simulink model "BVH2_App_Layer"  (Simulink 5.1)
settings: Solver=ode45  StartTime=0.0  StopTime=10.0  RelTol=1e-3
PreLoadFcn:
  | if exist('tl_preloadfcn','file'), tl_preloadfcn(gcs,95); end
PostLoadFcn:
  | if exist('tl_postloadfcn','file'), tl_postloadfcn(gcs,95); end
InitFcn:
  | if exist('tlds_start','file'), tlds_start(gcs); end
undefined symbols (not defined in the file): built, constant, Constant, DiscreteIntegrator, Gain, in, Logic, Product, Saturate, Sum, Switch
libraries: tllib x71, simulink x1
(part 2 of 4)

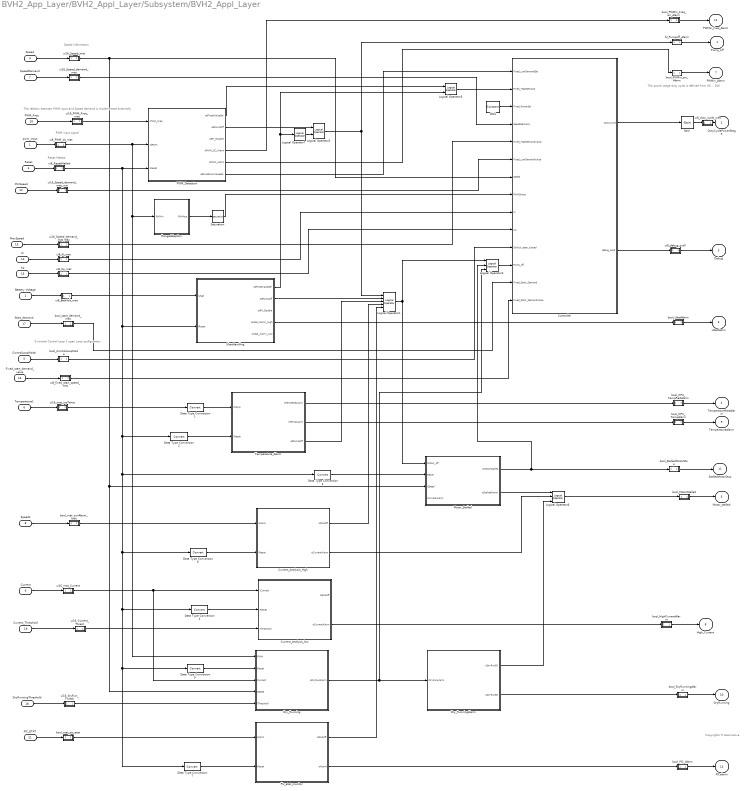
== system BVH2_App_Layer/BVH2_Appl_Layer/Subsystem/BVH2_Appl_Layer ==
  note: Copyrights
      | TI Automotive
  note: The power stage duty cycle
      | is defined from 00 .. 200
  note: 0   normal Control Loop
      | 1 open Loop configuration
  note: The relation between PWM input
      | and Speed demand is implemented externally
  note: Speed information
  note: PWM input signal
  note: Reset Matlab
  pwm_input : Inport  PortDimensions=1  SampleTime=0.01
      settings: CopyFcn=if exist('tl_check_ports','file'), tl_check_ports(gcbh); end  NameChangeFcn=if exist('tl_check_ports','file'), tl_check_ports(gcbh); end
  Battery Voltage : Inport  Port=2  PortDimensions=1  SampleTime=0.01
      settings: CopyFcn=if exist('tl_check_ports','file'), tl_check_ports(gcbh); end  NameChangeFcn=if exist('tl_check_ports','file'), tl_check_ports(gcbh); end
  Reset : Inport  Port=3  SampleTime=0.01
      settings: CopyFcn=if exist('tl_check_ports','file'), tl_check_ports(gcbh); end  NameChangeFcn=if exist('tl_check_ports','file'), tl_check_ports(gcbh); end
  Speed : Inport  Port=4  PortDimensions=1  SampleTime=0.01
      settings: CopyFcn=if exist('tl_check_ports','file'), tl_check_ports(gcbh); end  NameChangeFcn=if exist('tl_check_ports','file'), tl_check_ports(gcbh); end
  ControlLoopMode : Inport  Port=5  PortDimensions=1  SampleTime=0.01
      settings: CopyFcn=if exist('tl_check_ports','file'), tl_check_ports(gcbh); end  NameChangeFcn=if exist('tl_check_ports','file'), tl_check_ports(gcbh); end
  Temperature1 : Inport  Port=6  PortDimensions=1  SampleTime=0.01
      settings: CopyFcn=if exist('tl_check_ports','file'), tl_check_ports(gcbh); end  NameChangeFcn=if exist('tl_check_ports','file'), tl_check_ports(gcbh); end
  SpeedDemand : Inport  Port=7  PortDimensions=1  SampleTime=0.01
      settings: CopyFcn=if exist('tl_check_ports','file'), tl_check_ports(gcbh); end  NameChangeFcn=if exist('tl_check_ports','file'), tl_check_ports(gcbh); end
  Speed1 : Inport  Port=8  PortDimensions=1  SampleTime=0.01
      settings: CopyFcn=if exist('tl_check_ports','file'), tl_check_ports(gcbh); end  NameChangeFcn=if exist('tl_check_ports','file'), tl_check_ports(gcbh); end
  Current : Inport  Port=9  PortDimensions=1  SampleTime=0.01
      settings: CopyFcn=if exist('tl_check_ports','file'), tl_check_ports(gcbh); end  NameChangeFcn=if exist('tl_check_ports','file'), tl_check_ports(gcbh); end
  PWM_Freq : Inport  Port=10  PortDimensions=1  SampleTime=0.01
      settings: CopyFcn=if exist('tl_check_ports','file'), tl_check_ports(gcbh); end  NameChangeFcn=if exist('tl_check_ports','file'), tl_check_ports(gcbh); end
  PIC_ETAT : Inport  Port=11  PortDimensions=1  SampleTime=0.01
      settings: CopyFcn=if exist('tl_check_ports','file'), tl_check_ports(gcbh); end  NameChangeFcn=if exist('tl_check_ports','file'), tl_check_ports(gcbh); end
  MinSpeed : Inport  Port=12  SampleTime=0.01
      settings: CopyFcn=if exist('tl_check_ports','file'), tl_check_ports(gcbh); end  NameChangeFcn=if exist('tl_check_ports','file'), tl_check_ports(gcbh); end
  MaxSpeed : Inport  Port=13  SampleTime=0.01
      settings: CopyFcn=if exist('tl_check_ports','file'), tl_check_ports(gcbh); end  NameChangeFcn=if exist('tl_check_ports','file'), tl_check_ports(gcbh); end
  Ki : Inport  Port=14  SampleTime=0.01
      settings: CopyFcn=if exist('tl_check_ports','file'), tl_check_ports(gcbh); end  NameChangeFcn=if exist('tl_check_ports','file'), tl_check_ports(gcbh); end
  Kp : Inport  Port=15  SampleTime=0.01
      settings: CopyFcn=if exist('tl_check_ports','file'), tl_check_ports(gcbh); end  NameChangeFcn=if exist('tl_check_ports','file'), tl_check_ports(gcbh); end
  Fixed_start_demand_value : Inport  Port=16  PortDimensions=1  SampleTime=0.01
      settings: CopyFcn=if exist('tl_check_ports','file'), tl_check_ports(gcbh); end  NameChangeFcn=if exist('tl_check_ports','file'), tl_check_ports(gcbh); end
  Start_demand : Inport  Port=17  PortDimensions=1  SampleTime=0.01
      settings: CopyFcn=if exist('tl_check_ports','file'), tl_check_ports(gcbh); end  NameChangeFcn=if exist('tl_check_ports','file'), tl_check_ports(gcbh); end
  DryRunningThreshold : Inport  Port=18  PortDimensions=1  SampleTime=0.01
      settings: CopyFcn=if exist('tl_check_ports','file'), tl_check_ports(gcbh); end  NameChangeFcn=if exist('tl_check_ports','file'), tl_check_ports(gcbh); end
  Current_Threshold : Inport  Port=19  PortDimensions=1  SampleTime=0.01
      settings: CopyFcn=if exist('tl_check_ports','file'), tl_check_ports(gcbh); end  NameChangeFcn=if exist('tl_check_ports','file'), tl_check_ports(gcbh); end
  Controller : Subsystem
  Current_Analysis_High : Stateflow chart
  Current_Analysis_low : Stateflow chart
  Data Type Conversion{1..7} (7 alike) : DataTypeConversion  SaturateOnIntegerOverflow=on
  Dry_Running : Stateflow chart
  Dry_RunningAlarm : Stateflow chart
  Gain : tllib/Gain  data=struct('comment',struct('text','','placement',1),'logdata',struct('maxnumvals',inf,'plotchannels',[],'loggingmode',3,'channels',1),'output',struct('variable','','description','','name','$S_$B','width',1,'address','','max',NaN,'min',NaN,'class','default','type','Int16','scaling','','lsb',1,'offset',0,'arb',0,'freeze',1,'unit','','autoscalingmode',1,'lowerheadroom',1,'upperheadroom',1,'headroomunit','bit','keepdatatype',1,'checkmin',0,'checkmax',0,'castoutput',0,'show',0),'gain',struct('variable','','description','','name','$S_$B_gain','width',1,'address','','max',NaN,'min',NaN,'class','default','type','Int16','scaling','','lsb',1,'offset',0,'arb',0,'freeze',1,'unit','','keepdatatype',1,'value','0.5','scalar',0,'tolerance',1),'scalingvalid',0,'date',734649.702698634)  gain=0.5  flp_block=built-in/Gain
  Logical Operator1 : tllib/Logical Operator  data=struct('inputs','5','comment',struct('text','','placement',1),'logdata',struct('maxnumvals',inf,'plotchannels',[],'loggingmode',3,'channels',1),'operator','OR','output',struct('variable','','description','','name','$S_$B','address','','class','default','type','Bool','unit',''),'scalingvalid',0,'date',736089.717150243)  flp_block=built-in/Logic
  Logical Operator2 : tllib/Logical Operator  data=struct('inputs','2','comment',struct('text','','placement',1),'logdata',struct('maxnumvals',inf,'plotchannels',[],'loggingmode',3,'channels',1),'operator','AND','output',struct('variable','','description','','name','$S_$B','address','','class','default','type','Bool','unit',''),'scalingvalid',0,'date',735166.438757674)  flp_block=built-in/Logic
  Logical Operator3 : tllib/Logical Operator  data=struct('inputs','3','comment',struct('text','','placement',1),'logdata',struct('maxnumvals',inf,'plotchannels',[],'loggingmode',3,'channels',1),'operator','OR','output',struct('variable','','description','','name','$S_$B','address','','class','default','type','Bool','unit',''),'scalingvalid',0,'date',736089.716464456)  flp_block=built-in/Logic
  Logical Operator5 : tllib/Logical Operator  data=struct('inputs','2','comment',struct('text','','placement',1),'logdata',struct('maxnumvals',inf,'plotchannels',[],'loggingmode',3,'channels',1),'operator','OR','output',struct('variable','','description','','name','$S_$B','address','','class','default','type','Bool','unit',''),'scalingvalid',0,'date',735166.427160579)  flp_block=built-in/Logic
  Logical Operator6 : tllib/Logical Operator  data=struct('inputs','3','comment',struct('text','','placement',1),'logdata',struct('maxnumvals',inf,'plotchannels',[],'loggingmode',3,'channels',1),'operator','OR','output',struct('variable','','description','','name','$S_$B','address','','class','default','type','Bool','unit',''),'scalingvalid',0,'date',736074.585590822)  flp_block=built-in/Logic
  Logical Operator7 : tllib/Logical Operator  data=struct('inputs','1','comment',struct('text','','placement',1),'logdata',struct('maxnumvals',inf,'plotchannels',[],'loggingmode',3,'channels',1),'operator','NOT','output',struct('variable','','description','','name','$S_$B','address','','class','default','type','Bool','unit',''),'scalingvalid',0,'date',735166.438991285)  flp_block=built-in/Logic
  Motor_Stalled : Stateflow chart
  ON4 : tllib/Constant  Value=constant  ShowAdditionalParam=off  OutDataType=sfix(16)  ConRadixGroup=Use specified scaling  OutScaling=2^0  data=struct('comment',struct('text','','placement',1),'output',struct('width',1,'name','$S_$B','unit','','type','Int16','offset',0,'max',NaN,'min',NaN,'freeze',1,'lsb',1,'arb',0,'class','default','address','','description','','value','0','tolerance',1,'show',0,'variable','','scaling','','keepdatatype',1),'date',734769.5812564,'scalingvalid',0)  constant=0  flp_block=built-in/Constant  help=|
      | Constant block of dSPACE TargetLink.
      | 
      | Output signal keeps the given constant value.
  PWM_Detection : Stateflow chart
  Pic_etat_monitor : Stateflow chart
  RangeAdaption : Subsystem
  Saturation : tllib/Saturation  data=struct('comment',struct('text','','placement',1),'logdata',struct('maxnumvals',inf,'plotchannels',[],'loggingmode',3,'channels',1),'output',struct('variable','','description','','name','$S_$B','width',1,'address','','max',NaN,'min',NaN,'class','default','type','UInt8','scaling','','lsb',1,'offset',0,'arb',0,'freeze',1,'unit','','autoscalingmode',1,'lowerheadroom',0,'upperheadroom',1,'headroomunit','bit','keepdatatype',1,'castoutput',0,'show',0),'lowerlimit',struct('variable','','description','','name','$S_$B_lower','width',1,'address','','max',NaN,'min',NaN,'class','default','type','Int16','scaling','','lsb',1,'offset',0,'arb',0,'freeze',1,'unit','','keepdatatype',1,'value','60','scalar',0),'upperlimit',struct('variable','','description','','name','$S_$B_upper','width',1,'address','','max',NaN,'min',NaN,'class','default','type','Int16','scaling','','lsb',1,'offset',0,'arb',0,'freeze',1,'unit','','keepdatatype',1,'value','200','scalar',0),'scalingvalid',0,'date',734975.431625949)  lower_limit=60  upper_limit=200  flp_block=built-in/Saturate
  Temperature_Alarm : Stateflow chart
  UbatHandling : Stateflow chart
  bl_Pumpoff_Alarm : Subsystem  BlockChoice=Virtual  mask(TL_Outport){data=struct('comment',struct('text','','placement',1),'logdata',struct('maxnumvals',inf,'plotchannels',[],'loggingmode',3,'channels',1),'output',struct('width',1,'name','$B','unit','','type','Bool','offset',0,'max',NaN,'min',NaN,'freeze',1,'lsb',1,'arb',0,'class','GLOBAL','address','','description','','autoscalingmode',1,'lowerheadroom',0,'upperheadroom',1,'headroomunit','bit','checkmin',0,'checkmax',0,'show',0,'variable','','scaling','','keepdatatype',1,'castoutput',0),'date',734767.568817153,'message',struct('name','','component',''),'virtual',1,'scalingvalid',0), flp_block=none, slscaleparams=, help=|}
      mask help=|
      | OutPort block of dSPACE TargetLink.
      |
      | Input signal is scaled:
      |
      |         y = lsb * u + offset
      mask help:
      | TargetLink Outport block:
      | Defines the output interface of a TargetLink subsystem.
      mask init:
      | tlData = eval(data);
      | w = tlData.output.width;
      | if ~isempty(tlData.output.variable)
      |    [bExist,hVar] = dsdd('Exist',['/Pool/Variables/' tlData.output.variable],'ObjectKind','Variable');
      |    if bExist,
      |       w = dsdd('GetWidth',hVar);
      |       if isempty(w)
      |          w = 1;
      |       end
      |    end
      | end
      | if ~strcmp(get_param(gcbh,'TemplateBlock'),'')
      |    if tlData.virtual,
      |       if tlData.logdata.loggingmode == 3
      |          set_param(gcbh,'BlockChoice','Virtual');
      |       else
      |          set_param(gcbh,'BlockChoice','Mixed');
      |       end
      |    else
      |       set_param(gcbh,'BlockChoice','NonVirtual');
      |    end
      | end
      | clear tlData
      settings: DeleteFcn=delete_tlblock(gcbh);  NameChangeFcn=rename_tlblock(gcbh);  OpenFcn=dstabdlg('create','tl_port_dlg',gcbh);  TemplateBlock=tllib/OutPort  MemberBlocks=Mixed,NonVirtual,Virtual
      mask Help: eval(['tl_online_help(''Topic'',''',get_param(gcbh,'MaskType'),''')'])
      mask Display: plot([0 .2 .2 .8 .8; 1 .8 .8 .8 .8],[.5 .6 .4 .6 .4;.5 .6 .4 .8 .2]);
  bool_CPU_TempAlarm : Subsystem  BlockChoice=Virtual  mask(TL_Outport){data=struct('comment',struct('text','','placement',1),'logdata',struct('maxnumvals',inf,'plotchannels',[],'loggingmode',3,'channels',1),'output',struct('width',1,'name','$B','unit','','type','Bool','offset',0,'max',NaN,'min',NaN,'freeze',1,'lsb',1,'arb',0,'class','GLOBAL','address','','description','','autoscalingmode',1,'lowerheadroom',0,'upperheadroom',1,'headroomunit','bit','checkmin',0,'checkmax',0,'show',0,'variable','','scaling','','keepdatatype',1,'castoutput',0),'date',734773.577754271,'message',struct('name','','component',''),'virtual',1,'scalingvalid',0), flp_block=none, slscaleparams=, help=|}
      mask help=|
      | OutPort block of dSPACE TargetLink.
      |
      | Input signal is scaled:
      |
      |         y = lsb * u + offset
      mask help:
      | TargetLink Outport block:
      | Defines the output interface of a TargetLink subsystem.
      mask init: same as BVH2_App_Layer/BVH2_Appl_Layer/Subsystem/BVH2_Appl_Layer/bl_Pumpoff_Alarm
      settings: DeleteFcn=delete_tlblock(gcbh);  NameChangeFcn=rename_tlblock(gcbh);  OpenFcn=dstabdlg('create','tl_port_dlg',gcbh);  TemplateBlock=tllib/OutPort  MemberBlocks=Mixed,NonVirtual,Virtual
      mask Help: eval(['tl_online_help(''Topic'',''',get_param(gcbh,'MaskType'),''')'])
      mask Display: plot([0 .2 .2 .8 .8; 1 .8 .8 .8 .8],[.5 .6 .4 .6 .4;.5 .6 .4 .8 .2]);
  bool_CPU_TempRedAlarm : Subsystem  BlockChoice=Virtual  mask(TL_Outport){data=struct('comment',struct('text','','placement',1),'logdata',struct('maxnumvals',inf,'plotchannels',[],'loggingmode',3,'channels',1),'output',struct('width',1,'name','$B','unit','','type','Bool','offset',0,'max',NaN,'min',NaN,'freeze',1,'lsb',1,'arb',0,'class','GLOBAL','address','','description','','autoscalingmode',1,'lowerheadroom',0,'upperheadroom',1,'headroomunit','bit','checkmin',0,'checkmax',0,'show',0,'variable','','scaling','','keepdatatype',1,'castoutput',0),'date',734773.577754271,'message',struct('name','','component',''),'virtual',1,'scalingvalid',0), flp_block=none, slscaleparams=, help=|}
      mask help=|
      | OutPort block of dSPACE TargetLink.
      |
      | Input signal is scaled:
      |
      |         y = lsb * u + offset
      mask help:
      | TargetLink Outport block:
      | Defines the output interface of a TargetLink subsystem.
      mask init: same as BVH2_App_Layer/BVH2_Appl_Layer/Subsystem/BVH2_Appl_Layer/bl_Pumpoff_Alarm
      settings: DeleteFcn=delete_tlblock(gcbh);  NameChangeFcn=rename_tlblock(gcbh);  OpenFcn=dstabdlg('create','tl_port_dlg',gcbh);  TemplateBlock=tllib/OutPort  MemberBlocks=Mixed,NonVirtual,Virtual
      mask Help: eval(['tl_online_help(''Topic'',''',get_param(gcbh,'MaskType'),''')'])
      mask Display: plot([0 .2 .2 .8 .8; 1 .8 .8 .8 .8],[.5 .6 .4 .6 .4;.5 .6 .4 .8 .2]);
  bool_ControlLoopMode : Subsystem  BlockChoice=Mixed  mask(TL_Inport){data=struct('logdata',struct('maxnumvals',inf,'plotchannels',1,'loggingmode',1,'channels',1),'output',struct('width',1,'name','$B','unit','','type','Bool','offset',0,'max',NaN,'min',NaN,'freeze',1,'lsb',1,'arb',0,'class','GLOBAL','address','','description','','autoscalingmode',1,'lowerheadroom',0,'upperheadroom',1,'headroomunit','bit','show',0,'variable','','scaling','','keepdatatype',1,'castoutput',0),'date',734773.443896898,'message',struct('name','','component','','accessor',''),'virtual',1,'scalingvalid',0), flp_block=none, slscaleparams=, help=|}
      mask help=|
      | InPort block of dSPACE TargetLink.
      |
      | Input signal is read from an external variable and scaled:
      |
      |         y = lsb * u + offset
      mask help:
      | TargetLink Inport block:
      | Defines the input interface of a TargetLink subsystem.
      mask init: same as BVH2_App_Layer/BVH2_Appl_Layer/Subsystem/BVH2_Appl_Layer/bl_Pumpoff_Alarm
      settings: DeleteFcn=delete_tlblock(gcbh);  NameChangeFcn=rename_tlblock(gcbh);  OpenFcn=dstabdlg('create','tl_port_dlg',gcbh);  TemplateBlock=tllib/InPort  MemberBlocks=Mixed,NonVirtual,Virtual
      mask Help: eval(['tl_online_help(''Topic'',''',get_param(gcbh,'MaskType'),''')'])
      mask Display: plot([.2 0 .2 .2 .2;.2 1 .8 .8 .2],[.8 .5 .6 .4 .2;.6 .5 .6 .4 .4]);
  bool_DryRunningAlarm : Subsystem  BlockChoice=Virtual  mask(TL_Outport){data=struct('comment',struct('text','','placement',1),'logdata',struct('maxnumvals',inf,'plotchannels',[],'loggingmode',3,'channels',1),'output',struct('width',1,'name','$B','unit','','type','Bool','offset',0,'max',NaN,'min',NaN,'freeze',1,'lsb',1,'arb',0,'class','GLOBAL','address','','description','','autoscalingmode',1,'lowerheadroom',0,'upperheadroom',1,'headroomunit','bit','checkmin',0,'checkmax',0,'show',0,'variable','','scaling','','keepdatatype',1,'castoutput',0),'date',734773.60810485,'message',struct('name','','component',''),'virtual',1,'scalingvalid',0), flp_block=none, slscaleparams=, help=|}
      mask help=|
      | OutPort block of dSPACE TargetLink.
      |
      | Input signal is scaled:
      |
      |         y = lsb * u + offset
      mask help:
      | TargetLink Outport block:
      | Defines the output interface of a TargetLink subsystem.
      mask init: same as BVH2_App_Layer/BVH2_Appl_Layer/Subsystem/BVH2_Appl_Layer/bl_Pumpoff_Alarm
      settings: DeleteFcn=delete_tlblock(gcbh);  NameChangeFcn=rename_tlblock(gcbh);  OpenFcn=dstabdlg('create','tl_port_dlg',gcbh);  TemplateBlock=tllib/OutPort  MemberBlocks=Mixed,NonVirtual,Virtual
      mask Help: eval(['tl_online_help(''Topic'',''',get_param(gcbh,'MaskType'),''')'])
      mask Display: plot([0 .2 .2 .8 .8; 1 .8 .8 .8 .8],[.5 .6 .4 .6 .4;.5 .6 .4 .8 .2]);
  bool_HighCurrentAlarm : Subsystem  BlockChoice=Virtual  mask(TL_Outport){data=struct('comment',struct('text','','placement',1),'logdata',struct('maxnumvals',inf,'plotchannels',[],'loggingmode',3,'channels',1),'output',struct('width',1,'name','$B','unit','','type','Bool','offset',0,'max',NaN,'min',NaN,'freeze',1,'lsb',1,'arb',0,'class','GLOBAL','address','','description','','autoscalingmode',1,'lowerheadroom',0,'upperheadroom',1,'headroomunit','bit','checkmin',0,'checkmax',0,'show',0,'variable','','scaling','','keepdatatype',1,'castoutput',0),'date',734773.60810485,'message',struct('name','','component',''),'virtual',1,'scalingvalid',0), flp_block=none, slscaleparams=, help=|}
      mask help=|
      | OutPort block of dSPACE TargetLink.
      |
      | Input signal is scaled:
      |
      |         y = lsb * u + offset
      mask help:
      | TargetLink Outport block:
      | Defines the output interface of a TargetLink subsystem.
      mask init: same as BVH2_App_Layer/BVH2_Appl_Layer/Subsystem/BVH2_Appl_Layer/bl_Pumpoff_Alarm
      settings: DeleteFcn=delete_tlblock(gcbh);  NameChangeFcn=rename_tlblock(gcbh);  OpenFcn=dstabdlg('create','tl_port_dlg',gcbh);  TemplateBlock=tllib/OutPort  MemberBlocks=Mixed,NonVirtual,Virtual
      mask Help: eval(['tl_online_help(''Topic'',''',get_param(gcbh,'MaskType'),''')'])
      mask Display: plot([0 .2 .2 .8 .8; 1 .8 .8 .8 .8],[.5 .6 .4 .6 .4;.5 .6 .4 .8 .2]);
  bool_MotorStalled : Subsystem  BlockChoice=Virtual  mask(TL_Outport){data=struct('comment',struct('text','','placement',1),'logdata',struct('maxnumvals',inf,'plotchannels',[],'loggingmode',3,'channels',1),'output',struct('width',1,'name','$B','unit','','type','Bool','offset',0,'max',NaN,'min',NaN,'freeze',1,'lsb',1,'arb',0,'class','GLOBAL','address','','description','','autoscalingmode',1,'lowerheadroom',0,'upperheadroom',1,'headroomunit','bit','checkmin',0,'checkmax',0,'show',0,'variable','','scaling','','keepdatatype',1,'castoutput',0),'date',734773.60810485,'message',struct('name','','component',''),'virtual',1,'scalingvalid',0), flp_block=none, slscaleparams=, help=|}
      mask help=|
      | OutPort block of dSPACE TargetLink.
      |
      | Input signal is scaled:
      |
      |         y = lsb * u + offset
      mask help:
      | TargetLink Outport block:
      | Defines the output interface of a TargetLink subsystem.
      mask init: same as BVH2_App_Layer/BVH2_Appl_Layer/Subsystem/BVH2_Appl_Layer/bl_Pumpoff_Alarm
      settings: DeleteFcn=delete_tlblock(gcbh);  NameChangeFcn=rename_tlblock(gcbh);  OpenFcn=dstabdlg('create','tl_port_dlg',gcbh);  TemplateBlock=tllib/OutPort  MemberBlocks=Mixed,NonVirtual,Virtual
      mask Help: eval(['tl_online_help(''Topic'',''',get_param(gcbh,'MaskType'),''')'])
      mask Display: plot([0 .2 .2 .8 .8; 1 .8 .8 .8 .8],[.5 .6 .4 .6 .4;.5 .6 .4 .8 .2]);
  bool_PIC_Alarm : Subsystem  BlockChoice=Virtual  mask(TL_Outport){data=struct('comment',struct('text','','placement',1),'logdata',struct('maxnumvals',inf,'plotchannels',[],'loggingmode',3,'channels',1),'output',struct('width',1,'name','$B','unit','','type','Bool','offset',0,'max',NaN,'min',NaN,'freeze',1,'lsb',1,'arb',0,'class','GLOBAL','address','','description','','autoscalingmode',1,'lowerheadroom',0,'upperheadroom',1,'headroomunit','bit','checkmin',0,'checkmax',0,'show',0,'variable','','scaling','','keepdatatype',1,'castoutput',0),'date',734773.60810485,'message',struct('name','','component',''),'virtual',1,'scalingvalid',0), flp_block=none, slscaleparams=, help=|}
      mask help=|
      | OutPort block of dSPACE TargetLink.
      |
      | Input signal is scaled:
      |
      |         y = lsb * u + offset
      mask help:
      | TargetLink Outport block:
      | Defines the output interface of a TargetLink subsystem.
      mask init: same as BVH2_App_Layer/BVH2_Appl_Layer/Subsystem/BVH2_Appl_Layer/bl_Pumpoff_Alarm
      settings: DeleteFcn=delete_tlblock(gcbh);  NameChangeFcn=rename_tlblock(gcbh);  OpenFcn=dstabdlg('create','tl_port_dlg',gcbh);  TemplateBlock=tllib/OutPort  MemberBlocks=Mixed,NonVirtual,Virtual
      mask Help: eval(['tl_online_help(''Topic'',''',get_param(gcbh,'MaskType'),''')'])
      mask Display: plot([0 .2 .2 .8 .8; 1 .8 .8 .8 .8],[.5 .6 .4 .6 .4;.5 .6 .4 .8 .2]);
  bool_PWMin_Freq_err_Alarm : Subsystem  BlockChoice=Virtual  mask(TL_Outport){data=struct('comment',struct('text','','placement',1),'logdata',struct('maxnumvals',inf,'plotchannels',[],'loggingmode',3,'channels',1),'output',struct('width',1,'name','$B','unit','','type','Bool','offset',0,'max',NaN,'min',NaN,'freeze',1,'lsb',1,'arb',0,'class','GLOBAL','address','','description','','autoscalingmode',1,'lowerheadroom',0,'upperheadroom',1,'headroomunit','bit','checkmin',0,'checkmax',0,'show',0,'variable','','scaling','','keepdatatype',1,'castoutput',0),'date',734767.568817153,'message',struct('name','','component',''),'virtual',1,'scalingvalid',0), flp_block=none, slscaleparams=, help=|}
      mask help=|
      | OutPort block of dSPACE TargetLink.
      |
      | Input signal is scaled:
      |
      |         y = lsb * u + offset
      mask help:
      | TargetLink Outport block:
      | Defines the output interface of a TargetLink subsystem.
      mask init: same as BVH2_App_Layer/BVH2_Appl_Layer/Subsystem/BVH2_Appl_Layer/bl_Pumpoff_Alarm
      settings: DeleteFcn=delete_tlblock(gcbh);  NameChangeFcn=rename_tlblock(gcbh);  OpenFcn=dstabdlg('create','tl_port_dlg',gcbh);  TemplateBlock=tllib/OutPort  MemberBlocks=Mixed,NonVirtual,Virtual
      mask Help: eval(['tl_online_help(''Topic'',''',get_param(gcbh,'MaskType'),''')'])
      mask Display: plot([0 .2 .2 .8 .8; 1 .8 .8 .8 .8],[.5 .6 .4 .6 .4;.5 .6 .4 .8 .2]);
  bool_PWMin_err_Alarm : Subsystem  BlockChoice=Virtual  mask(TL_Outport){data=struct('comment',struct('text','','placement',1),'logdata',struct('maxnumvals',inf,'plotchannels',[],'loggingmode',3,'channels',1),'output',struct('width',1,'name','$B','unit','','type','Bool','offset',0,'max',NaN,'min',NaN,'freeze',1,'lsb',1,'arb',0,'class','GLOBAL','address','','description','','autoscalingmode',1,'lowerheadroom',0,'upperheadroom',1,'headroomunit','bit','checkmin',0,'checkmax',0,'show',0,'variable','','scaling','','keepdatatype',1,'castoutput',0),'date',734767.568817153,'message',struct('name','','component',''),'virtual',1,'scalingvalid',0), flp_block=none, slscaleparams=, help=|}
      mask help=|
      | OutPort block of dSPACE TargetLink.
      |
      | Input signal is scaled:
      |
      |         y = lsb * u + offset
      mask help:
      | TargetLink Outport block:
      | Defines the output interface of a TargetLink subsystem.
      mask init: same as BVH2_App_Layer/BVH2_Appl_Layer/Subsystem/BVH2_Appl_Layer/bl_Pumpoff_Alarm
      settings: DeleteFcn=delete_tlblock(gcbh);  NameChangeFcn=rename_tlblock(gcbh);  OpenFcn=dstabdlg('create','tl_port_dlg',gcbh);  TemplateBlock=tllib/OutPort  MemberBlocks=Mixed,NonVirtual,Virtual
      mask Help: eval(['tl_online_help(''Topic'',''',get_param(gcbh,'MaskType'),''')'])
      mask Display: plot([0 .2 .2 .8 .8; 1 .8 .8 .8 .8],[.5 .6 .4 .6 .4;.5 .6 .4 .8 .2]);
  bool_StalledMotorStop : Subsystem  BlockChoice=Virtual  mask(TL_Outport){data=struct('comment',struct('text','','placement',1),'logdata',struct('maxnumvals',inf,'plotchannels',[],'loggingmode',3,'channels',1),'output',struct('width',1,'name','$B','unit','','type','Bool','offset',0,'max',NaN,'min',NaN,'freeze',1,'lsb',1,'arb',0,'class','GLOBAL','address','','description','','autoscalingmode',1,'lowerheadroom',0,'upperheadroom',1,'headroomunit','bit','checkmin',0,'checkmax',0,'show',0,'variable','','scaling','','keepdatatype',1,'castoutput',0),'date',734773.60810485,'message',struct('name','','component',''),'virtual',1,'scalingvalid',0), flp_block=none, slscaleparams=, help=|}
      mask help=|
      | OutPort block of dSPACE TargetLink.
      |
      | Input signal is scaled:
      |
      |         y = lsb * u + offset
      mask help:
      | TargetLink Outport block:
      | Defines the output interface of a TargetLink subsystem.
      mask init: same as BVH2_App_Layer/BVH2_Appl_Layer/Subsystem/BVH2_Appl_Layer/bl_Pumpoff_Alarm
      settings: DeleteFcn=delete_tlblock(gcbh);  NameChangeFcn=rename_tlblock(gcbh);  OpenFcn=dstabdlg('create','tl_port_dlg',gcbh);  TemplateBlock=tllib/OutPort  MemberBlocks=Mixed,NonVirtual,Virtual
      mask Help: eval(['tl_online_help(''Topic'',''',get_param(gcbh,'MaskType'),''')'])
      mask Display: plot([0 .2 .2 .8 .8; 1 .8 .8 .8 .8],[.5 .6 .4 .6 .4;.5 .6 .4 .8 .2]);
  bool_UbatAlarm : Subsystem  BlockChoice=Virtual  mask(TL_Outport){data=struct('comment',struct('text','','placement',1),'logdata',struct('maxnumvals',inf,'plotchannels',[],'loggingmode',3,'channels',1),'output',struct('width',1,'name','$B','unit','','type','Bool','offset',0,'max',NaN,'min',NaN,'freeze',1,'lsb',1,'arb',0,'class','GLOBAL','address','','description','','autoscalingmode',1,'lowerheadroom',0,'upperheadroom',1,'headroomunit','bit','checkmin',0,'checkmax',0,'show',0,'variable','','scaling','','keepdatatype',1,'castoutput',0),'date',734767.568817153,'message',struct('name','','component',''),'virtual',1,'scalingvalid',0), flp_block=none, slscaleparams=, help=|}
      mask help=|
      | OutPort block of dSPACE TargetLink.
      |
      | Input signal is scaled:
      |
      |         y = lsb * u + offset
      mask help:
      | TargetLink Outport block:
      | Defines the output interface of a TargetLink subsystem.
      mask init: same as BVH2_App_Layer/BVH2_Appl_Layer/Subsystem/BVH2_Appl_Layer/bl_Pumpoff_Alarm
      settings: DeleteFcn=delete_tlblock(gcbh);  NameChangeFcn=rename_tlblock(gcbh);  OpenFcn=dstabdlg('create','tl_port_dlg',gcbh);  TemplateBlock=tllib/OutPort  MemberBlocks=Mixed,NonVirtual,Virtual
      mask Help: eval(['tl_online_help(''Topic'',''',get_param(gcbh,'MaskType'),''')'])
      mask Display: plot([0 .2 .2 .8 .8; 1 .8 .8 .8 .8],[.5 .6 .4 .6 .4;.5 .6 .4 .8 .2]);
  bool_mat_currAlarm_bldc : Subsystem  BlockChoice=Mixed  mask(TL_Inport){data=struct('logdata',struct('maxnumvals',inf,'plotchannels',1,'loggingmode',1,'channels',1),'output',struct('width',1,'name','$B','unit','','type','Bool','offset',0,'max',NaN,'min',NaN,'freeze',1,'lsb',1,'arb',0,'class','GLOBAL','address','','description','','autoscalingmode',1,'lowerheadroom',0,'upperheadroom',1,'headroomunit','bit','show',0,'variable','','scaling','','keepdatatype',1,'castoutput',0),'date',734892.488347951,'message',struct('name','','component','','accessor',''),'virtual',1,'scalingvalid',0), flp_block=none, slscaleparams=, help=|}
      mask help=|
      | InPort block of dSPACE TargetLink.
      |
      | Input signal is read from an external variable and scaled:
      |
      |         y = lsb * u + offset
      mask help:
      | TargetLink Inport block:
      | Defines the input interface of a TargetLink subsystem.
      mask init: same as BVH2_App_Layer/BVH2_Appl_Layer/Subsystem/BVH2_Appl_Layer/bl_Pumpoff_Alarm
      settings: DeleteFcn=delete_tlblock(gcbh);  NameChangeFcn=rename_tlblock(gcbh);  OpenFcn=dstabdlg('create','tl_port_dlg',gcbh);  TemplateBlock=tllib/InPort  MemberBlocks=Mixed,NonVirtual,Virtual
      mask Help: eval(['tl_online_help(''Topic'',''',get_param(gcbh,'MaskType'),''')'])
      mask Display: plot([.2 0 .2 .2 .2;.2 1 .8 .8 .2],[.8 .5 .6 .4 .2;.6 .5 .6 .4 .4]);
  bool_mat_pic_etat : Subsystem  BlockChoice=Mixed  mask(TL_Inport){data=struct('logdata',struct('maxnumvals',inf,'plotchannels',1,'loggingmode',1,'channels',1),'output',struct('width',1,'name','$B','unit','','type','Bool','offset',0,'max',NaN,'min',NaN,'freeze',1,'lsb',1,'arb',0,'class','GLOBAL','address','','description','','autoscalingmode',1,'lowerheadroom',0,'upperheadroom',1,'headroomunit','bit','show',0,'variable','','scaling','','keepdatatype',1,'castoutput',0),'date',735046.472280162,'message',struct('name','','component','','accessor',''),'virtual',1,'scalingvalid',0), flp_block=none, slscaleparams=, help=|}
      mask help=|
      | InPort block of dSPACE TargetLink.
      |
      | Input signal is read from an external variable and scaled:
      |
      |         y = lsb * u + offset
      mask help:
      | TargetLink Inport block:
      | Defines the input interface of a TargetLink subsystem.
      mask init: same as BVH2_App_Layer/BVH2_Appl_Layer/Subsystem/BVH2_Appl_Layer/bl_Pumpoff_Alarm
      settings: DeleteFcn=delete_tlblock(gcbh);  NameChangeFcn=rename_tlblock(gcbh);  OpenFcn=dstabdlg('create','tl_port_dlg',gcbh);  TemplateBlock=tllib/InPort  MemberBlocks=Mixed,NonVirtual,Virtual
      mask Help: eval(['tl_online_help(''Topic'',''',get_param(gcbh,'MaskType'),''')'])
      mask Display: plot([.2 0 .2 .2 .2;.2 1 .8 .8 .2],[.8 .5 .6 .4 .2;.6 .5 .6 .4 .4]);
  bool_start_demand_mat : Subsystem  BlockChoice=Mixed  mask(TL_Inport){data=struct('logdata',struct('maxnumvals',inf,'plotchannels',1,'loggingmode',1,'channels',1),'output',struct('width',1,'name','$B','unit','','type','Bool','offset',0,'max',NaN,'min',NaN,'freeze',1,'lsb',1,'arb',0,'class','GLOBAL','address','','description','','autoscalingmode',1,'lowerheadroom',0,'upperheadroom',1,'headroomunit','bit','show',0,'variable','','scaling','','keepdatatype',1,'castoutput',0),'date',734773.443896898,'message',struct('name','','component','','accessor',''),'virtual',1,'scalingvalid',0), flp_block=none, slscaleparams=, help=|}
      mask help=|
      | InPort block of dSPACE TargetLink.
      |
      | Input signal is read from an external variable and scaled:
      |
      |         y = lsb * u + offset
      mask help:
      | TargetLink Inport block:
      | Defines the input interface of a TargetLink subsystem.
      mask init: same as BVH2_App_Layer/BVH2_Appl_Layer/Subsystem/BVH2_Appl_Layer/bl_Pumpoff_Alarm
      settings: DeleteFcn=delete_tlblock(gcbh);  NameChangeFcn=rename_tlblock(gcbh);  OpenFcn=dstabdlg('create','tl_port_dlg',gcbh);  TemplateBlock=tllib/InPort  MemberBlocks=Mixed,NonVirtual,Virtual
      mask Help: eval(['tl_online_help(''Topic'',''',get_param(gcbh,'MaskType'),''')'])
      mask Display: plot([.2 0 .2 .2 .2;.2 1 .8 .8 .2],[.8 .5 .6 .4 .2;.6 .5 .6 .4 .4]);
  ui16_Current_Thresh : Subsystem  BlockChoice=Mixed  mask(TL_Inport){data=struct('logdata',struct('maxnumvals',inf,'plotchannels',1,'loggingmode',1,'channels',1),'output',struct('width',1,'name','$B','unit','','type','UInt16','offset',0,'max',NaN,'min',NaN,'freeze',1,'lsb',1,'arb',0,'class','GLOBAL','address','','description','','autoscalingmode',1,'lowerheadroom',0,'upperheadroom',1,'headroomunit','bit','show',0,'variable','','scaling','','keepdatatype',1,'castoutput',0),'date',734773.690678611,'message',struct('name','','component','','accessor',''),'virtual',1,'scalingvalid',0), flp_block=none, slscaleparams=, help=|}
      mask help=|
      | InPort block of dSPACE TargetLink.
      |
      | Input signal is read from an external variable and scaled:
      |
      |         y = lsb * u + offset
      mask help:
      | TargetLink Inport block:
      | Defines the input interface of a TargetLink subsystem.
      mask init: same as BVH2_App_Layer/BVH2_Appl_Layer/Subsystem/BVH2_Appl_Layer/bl_Pumpoff_Alarm
      settings: DeleteFcn=delete_tlblock(gcbh);  NameChangeFcn=rename_tlblock(gcbh);  OpenFcn=dstabdlg('create','tl_port_dlg',gcbh);  TemplateBlock=tllib/InPort  MemberBlocks=Mixed,NonVirtual,Virtual
      mask Help: eval(['tl_online_help(''Topic'',''',get_param(gcbh,'MaskType'),''')'])
      mask Display: plot([.2 0 .2 .2 .2;.2 1 .8 .8 .2],[.8 .5 .6 .4 .2;.6 .5 .6 .4 .4]);
  ui16_PWM_Freq_mat : Subsystem  BlockChoice=Mixed  mask(TL_Inport){data=struct('logdata',struct('maxnumvals',inf,'plotchannels',1,'loggingmode',1,'channels',1),'output',struct('width',1,'name','$B','unit','','type','UInt16','offset',0,'max',200,'min',0,'freeze',1,'lsb',1,'arb',0,'class','GLOBAL','address','','description','','autoscalingmode',1,'lowerheadroom',0,'upperheadroom',1,'headroomunit','bit','show',0,'variable','','scaling','','keepdatatype',1,'castoutput',0),'date',734894.635327361,'message',struct('name','','component','','accessor',''),'virtual',1,'scalingvalid',0), flp_block=none, slscaleparams=, help=|}
      mask help=|
      | InPort block of dSPACE TargetLink.
      |
      | Input signal is read from an external variable and scaled:
      |
      |         y = lsb * u + offset
      mask help:
      | TargetLink Inport block:
      | Defines the input interface of a TargetLink subsystem.
      mask init: same as BVH2_App_Layer/BVH2_Appl_Layer/Subsystem/BVH2_Appl_Layer/bl_Pumpoff_Alarm
      settings: DeleteFcn=delete_tlblock(gcbh);  NameChangeFcn=rename_tlblock(gcbh);  OpenFcn=dstabdlg('create','tl_port_dlg',gcbh);  TemplateBlock=tllib/InPort  MemberBlocks=Mixed,NonVirtual,Virtual
      mask Help: eval(['tl_online_help(''Topic'',''',get_param(gcbh,'MaskType'),''')'])
      mask Display: plot([.2 0 .2 .2 .2;.2 1 .8 .8 .2],[.8 .5 .6 .4 .2;.6 .5 .6 .4 .4]);
  ui16_Speed_demand_mat : Subsystem  BlockChoice=Mixed  mask(TL_Inport){data=struct('logdata',struct('maxnumvals',inf,'plotchannels',1,'loggingmode',1,'channels',1),'output',struct('width',1,'name','$B','unit','','type','UInt16','offset',0,'max',200,'min',0,'freeze',1,'lsb',1,'arb',0,'class','GLOBAL','address','','description','','autoscalingmode',1,'lowerheadroom',0,'upperheadroom',1,'headroomunit','bit','show',0,'variable','','scaling','','keepdatatype',1,'castoutput',0),'date',734880.553248854,'message',struct('name','','component','','accessor',''),'virtual',1,'scalingvalid',0), flp_block=none, slscaleparams=, help=|}
      mask help=|
      | InPort block of dSPACE TargetLink.
      |
      | Input signal is read from an external variable and scaled:
      |
      |         y = lsb * u + offset
      mask help:
      | TargetLink Inport block:
      | Defines the input interface of a TargetLink subsystem.
      mask init: same as BVH2_App_Layer/BVH2_Appl_Layer/Subsystem/BVH2_Appl_Layer/bl_Pumpoff_Alarm
      settings: DeleteFcn=delete_tlblock(gcbh);  NameChangeFcn=rename_tlblock(gcbh);  OpenFcn=dstabdlg('create','tl_port_dlg',gcbh);  TemplateBlock=tllib/InPort  MemberBlocks=Mixed,NonVirtual,Virtual
      mask Help: eval(['tl_online_help(''Topic'',''',get_param(gcbh,'MaskType'),''')'])
      mask Display: plot([.2 0 .2 .2 .2;.2 1 .8 .8 .2],[.8 .5 .6 .4 .2;.6 .5 .6 .4 .4]);
  ui16_Speed_demand_mat_Max : Subsystem  BlockChoice=Mixed  mask(TL_Inport){data=struct('logdata',struct('maxnumvals',inf,'plotchannels',1,'loggingmode',1,'channels',1),'output',struct('width',1,'name','$B','unit','','type','UInt16','offset',0,'max',200,'min',0,'freeze',1,'lsb',1,'arb',0,'class','GLOBAL','address','','description','','autoscalingmode',1,'lowerheadroom',0,'upperheadroom',1,'headroomunit','bit','show',0,'variable','','scaling','','keepdatatype',1,'castoutput',0),'date',735054.434824826,'message',struct('name','','component','','accessor',''),'virtual',1,'scalingvalid',0), flp_block=none, slscaleparams=, help=|}
      mask help=|
      | InPort block of dSPACE TargetLink.
      |
      | Input signal is read from an external variable and scaled:
      |
      |         y = lsb * u + offset
      mask help:
      | TargetLink Inport block:
      | Defines the input interface of a TargetLink subsystem.
      mask init: same as BVH2_App_Layer/BVH2_Appl_Layer/Subsystem/BVH2_Appl_Layer/bl_Pumpoff_Alarm
      settings: DeleteFcn=delete_tlblock(gcbh);  NameChangeFcn=rename_tlblock(gcbh);  OpenFcn=dstabdlg('create','tl_port_dlg',gcbh);  TemplateBlock=tllib/InPort  MemberBlocks=Mixed,NonVirtual,Virtual
      mask Help: eval(['tl_online_help(''Topic'',''',get_param(gcbh,'MaskType'),''')'])
      mask Display: plot([.2 0 .2 .2 .2;.2 1 .8 .8 .2],[.8 .5 .6 .4 .2;.6 .5 .6 .4 .4]);
  ui16_Speed_demand_mat_min : Subsystem  BlockChoice=Mixed  mask(TL_Inport){data=struct('logdata',struct('maxnumvals',inf,'plotchannels',1,'loggingmode',1,'channels',1),'output',struct('width',1,'name','$B','unit','','type','UInt16','offset',0,'max',200,'min',0,'freeze',1,'lsb',1,'arb',0,'class','GLOBAL','address','','description','','autoscalingmode',1,'lowerheadroom',0,'upperheadroom',1,'headroomunit','bit','show',0,'variable','','scaling','','keepdatatype',1,'castoutput',0),'date',735054.43471831,'message',struct('name','','component','','accessor',''),'virtual',1,'scalingvalid',0), flp_block=none, slscaleparams=, help=|}
      mask help=|
      | InPort block of dSPACE TargetLink.
      |
      | Input signal is read from an external variable and scaled:
      |
      |         y = lsb * u + offset
      mask help:
      | TargetLink Inport block:
      | Defines the input interface of a TargetLink subsystem.
      mask init: same as BVH2_App_Layer/BVH2_Appl_Layer/Subsystem/BVH2_Appl_Layer/bl_Pumpoff_Alarm
      settings: DeleteFcn=delete_tlblock(gcbh);  NameChangeFcn=rename_tlblock(gcbh);  OpenFcn=dstabdlg('create','tl_port_dlg',gcbh);  TemplateBlock=tllib/InPort  MemberBlocks=Mixed,NonVirtual,Virtual
      mask Help: eval(['tl_online_help(''Topic'',''',get_param(gcbh,'MaskType'),''')'])
      mask Display: plot([.2 0 .2 .2 .2;.2 1 .8 .8 .2],[.8 .5 .6 .4 .2;.6 .5 .6 .4 .4]);
  ui16_Speed_mat : Subsystem  BlockChoice=Mixed  mask(TL_Inport){data=struct('logdata',struct('maxnumvals',inf,'plotchannels',1,'loggingmode',1,'channels',1),'output',struct('width',1,'name','$B','unit','','type','UInt16','offset',0,'max',200,'min',0,'freeze',1,'lsb',1,'arb',0,'class','GLOBAL','address','','description','','autoscalingmode',1,'lowerheadroom',0,'upperheadroom',1,'headroomunit','bit','show',0,'variable','','scaling','','keepdatatype',1,'castoutput',0),'date',734774.460309225,'message',struct('name','','component','','accessor',''),'virtual',1,'scalingvalid',0), flp_block=none, slscaleparams=, help=|}
      mask help=|
      | InPort block of dSPACE TargetLink.
      |
      | Input signal is read from an external variable and scaled:
      |
      |         y = lsb * u + offset
      mask help:
      | TargetLink Inport block:
      | Defines the input interface of a TargetLink subsystem.
      mask init: same as BVH2_App_Layer/BVH2_Appl_Layer/Subsystem/BVH2_Appl_Layer/bl_Pumpoff_Alarm
      settings: DeleteFcn=delete_tlblock(gcbh);  NameChangeFcn=rename_tlblock(gcbh);  OpenFcn=dstabdlg('create','tl_port_dlg',gcbh);  TemplateBlock=tllib/InPort  MemberBlocks=Mixed,NonVirtual,Virtual
      mask Help: eval(['tl_online_help(''Topic'',''',get_param(gcbh,'MaskType'),''')'])
      mask Display: plot([.2 0 .2 .2 .2;.2 1 .8 .8 .2],[.8 .5 .6 .4 .2;.6 .5 .6 .4 .4]);
  ui16_dryRun_Thresh : Subsystem  BlockChoice=Mixed  mask(TL_Inport){data=struct('logdata',struct('maxnumvals',inf,'plotchannels',1,'loggingmode',1,'channels',1),'output',struct('width',1,'name','$B','unit','','type','UInt16','offset',0,'max',NaN,'min',NaN,'freeze',1,'lsb',1,'arb',0,'class','GLOBAL','address','','description','','autoscalingmode',1,'lowerheadroom',0,'upperheadroom',1,'headroomunit','bit','show',0,'variable','','scaling','','keepdatatype',1,'castoutput',0),'date',734773.690678611,'message',struct('name','','component','','accessor',''),'virtual',1,'scalingvalid',0), flp_block=none, slscaleparams=, help=|}
      mask help=|
      | InPort block of dSPACE TargetLink.
      |
      | Input signal is read from an external variable and scaled:
      |
      |         y = lsb * u + offset
      mask help:
      | TargetLink Inport block:
      | Defines the input interface of a TargetLink subsystem.
      mask init: same as BVH2_App_Layer/BVH2_Appl_Layer/Subsystem/BVH2_Appl_Layer/bl_Pumpoff_Alarm
      settings: DeleteFcn=delete_tlblock(gcbh);  NameChangeFcn=rename_tlblock(gcbh);  OpenFcn=dstabdlg('create','tl_port_dlg',gcbh);  TemplateBlock=tllib/InPort  MemberBlocks=Mixed,NonVirtual,Virtual
      mask Help: eval(['tl_online_help(''Topic'',''',get_param(gcbh,'MaskType'),''')'])
      mask Display: plot([.2 0 .2 .2 .2;.2 1 .8 .8 .2],[.8 .5 .6 .4 .2;.6 .5 .6 .4 .4]);
  ui16_mat_Current : Subsystem  BlockChoice=Mixed  mask(TL_Inport){data=struct('logdata',struct('maxnumvals',inf,'plotchannels',1,'loggingmode',1,'channels',1),'output',struct('width',1,'name','$B','unit','','type','UInt16','offset',0,'max',NaN,'min',NaN,'freeze',1,'lsb',1,'arb',0,'class','GLOBAL','address','','description','','autoscalingmode',1,'lowerheadroom',0,'upperheadroom',1,'headroomunit','bit','show',0,'variable','','scaling','','keepdatatype',1,'castoutput',0),'date',734773.690678611,'message',struct('name','','component','','accessor',''),'virtual',1,'scalingvalid',0), flp_block=none, slscaleparams=, help=|}
      mask help=|
      | InPort block of dSPACE TargetLink.
      |
      | Input signal is read from an external variable and scaled:
      |
      |         y = lsb * u + offset
      mask help:
      | TargetLink Inport block:
      | Defines the input interface of a TargetLink subsystem.
      mask init: same as BVH2_App_Layer/BVH2_Appl_Layer/Subsystem/BVH2_Appl_Layer/bl_Pumpoff_Alarm
      settings: DeleteFcn=delete_tlblock(gcbh);  NameChangeFcn=rename_tlblock(gcbh);  OpenFcn=dstabdlg('create','tl_port_dlg',gcbh);  TemplateBlock=tllib/InPort  MemberBlocks=Mixed,NonVirtual,Virtual
      mask Help: eval(['tl_online_help(''Topic'',''',get_param(gcbh,'MaskType'),''')'])
      mask Display: plot([.2 0 .2 .2 .2;.2 1 .8 .8 .2],[.8 .5 .6 .4 .2;.6 .5 .6 .4 .4]);
  ui16_mat_inpTemp : Subsystem  BlockChoice=Mixed  mask(TL_Inport){data=struct('logdata',struct('maxnumvals',inf,'plotchannels',1,'loggingmode',1,'channels',1),'output',struct('width',1,'name','$B','unit','','type','UInt16','offset',0,'max',NaN,'min',NaN,'freeze',1,'lsb',1,'arb',0,'class','GLOBAL','address','','description','','autoscalingmode',1,'lowerheadroom',0,'upperheadroom',1,'headroomunit','bit','show',0,'variable','','scaling','','keepdatatype',1,'castoutput',0),'date',734767.589264792,'message',struct('name','','component','','accessor',''),'virtual',1,'scalingvalid',0), flp_block=none, slscaleparams=, help=|}
      mask help=|
      | InPort block of dSPACE TargetLink.
      |
      | Input signal is read from an external variable and scaled:
      |
      |         y = lsb * u + offset
      mask help:
      | TargetLink Inport block:
      | Defines the input interface of a TargetLink subsystem.
      mask init: same as BVH2_App_Layer/BVH2_Appl_Layer/Subsystem/BVH2_Appl_Layer/bl_Pumpoff_Alarm
      settings: DeleteFcn=delete_tlblock(gcbh);  NameChangeFcn=rename_tlblock(gcbh);  OpenFcn=dstabdlg('create','tl_port_dlg',gcbh);  TemplateBlock=tllib/InPort  MemberBlocks=Mixed,NonVirtual,Virtual
      mask Help: eval(['tl_online_help(''Topic'',''',get_param(gcbh,'MaskType'),''')'])
      mask Display: plot([.2 0 .2 .2 .2;.2 1 .8 .8 .2],[.8 .5 .6 .4 .2;.6 .5 .6 .4 .4]);
  ui8_BattVolt_mat : Subsystem  BlockChoice=Mixed  mask(TL_Inport){data=struct('logdata',struct('maxnumvals',inf,'plotchannels',1,'loggingmode',1,'channels',1),'output',struct('width',1,'name','$B','unit','','type','UInt16','offset',0,'max',200,'min',0,'freeze',1,'lsb',1,'arb',0,'class','GLOBAL','address','','description','','autoscalingmode',1,'lowerheadroom',0,'upperheadroom',1,'headroomunit','bit','show',0,'variable','','scaling','','keepdatatype',1,'castoutput',0),'date',734692.64001684,'message',struct('name','','component','','accessor',''),'virtual',1,'scalingvalid',0), flp_block=none, slscaleparams=, help=|}
      mask help=|
      | InPort block of dSPACE TargetLink.
      |
      | Input signal is read from an external variable and scaled:
      |
      |         y = lsb * u + offset
      mask help:
      | TargetLink Inport block:
      | Defines the input interface of a TargetLink subsystem.
      mask init: same as BVH2_App_Layer/BVH2_Appl_Layer/Subsystem/BVH2_Appl_Layer/bl_Pumpoff_Alarm
      settings: DeleteFcn=delete_tlblock(gcbh);  NameChangeFcn=rename_tlblock(gcbh);  OpenFcn=dstabdlg('create','tl_port_dlg',gcbh);  TemplateBlock=tllib/InPort  MemberBlocks=Mixed,NonVirtual,Virtual
      mask Help: eval(['tl_online_help(''Topic'',''',get_param(gcbh,'MaskType'),''')'])
      mask Display: plot([.2 0 .2 .2 .2;.2 1 .8 .8 .2],[.8 .5 .6 .4 .2;.6 .5 .6 .4 .4]);
  ui8_Ki_mat : Subsystem  BlockChoice=Mixed  mask(TL_Inport){data=struct('logdata',struct('maxnumvals',inf,'plotchannels',1,'loggingmode',1,'channels',1),'output',struct('width',1,'name','$B','unit','','type','UInt16','offset',0,'max',200,'min',0,'freeze',1,'lsb',1,'arb',0,'class','GLOBAL','address','','description','','autoscalingmode',1,'lowerheadroom',0,'upperheadroom',1,'headroomunit','bit','show',0,'variable','','scaling','','keepdatatype',1,'castoutput',0),'date',735054.434824826,'message',struct('name','','component','','accessor',''),'virtual',1,'scalingvalid',0), flp_block=none, slscaleparams=, help=|}
      mask help=|
      | InPort block of dSPACE TargetLink.
      |
      | Input signal is read from an external variable and scaled:
      |
      |         y = lsb * u + offset
      mask help:
      | TargetLink Inport block:
      | Defines the input interface of a TargetLink subsystem.
      mask init: same as BVH2_App_Layer/BVH2_Appl_Layer/Subsystem/BVH2_Appl_Layer/bl_Pumpoff_Alarm
      settings: DeleteFcn=delete_tlblock(gcbh);  NameChangeFcn=rename_tlblock(gcbh);  OpenFcn=dstabdlg('create','tl_port_dlg',gcbh);  TemplateBlock=tllib/InPort  MemberBlocks=Mixed,NonVirtual,Virtual
      mask Help: eval(['tl_online_help(''Topic'',''',get_param(gcbh,'MaskType'),''')'])
      mask Display: plot([.2 0 .2 .2 .2;.2 1 .8 .8 .2],[.8 .5 .6 .4 .2;.6 .5 .6 .4 .4]);
  ui8_Kp_mat : Subsystem  BlockChoice=Mixed  mask(TL_Inport){data=struct('logdata',struct('maxnumvals',inf,'plotchannels',1,'loggingmode',1,'channels',1),'output',struct('width',1,'name','$B','unit','','type','UInt8','offset',0,'max',200,'min',0,'freeze',1,'lsb',1,'arb',0,'class','GLOBAL','address','','description','','autoscalingmode',1,'lowerheadroom',0,'upperheadroom',1,'headroomunit','bit','show',0,'variable','','scaling','','keepdatatype',1,'castoutput',0),'date',735188.475080671,'message',struct('name','','component','','accessor',''),'virtual',1,'scalingvalid',0), flp_block=none, slscaleparams=, help=|}
      mask help=|
      | InPort block of dSPACE TargetLink.
      |
      | Input signal is read from an external variable and scaled:
      |
      |         y = lsb * u + offset
      mask help:
      | TargetLink Inport block:
      | Defines the input interface of a TargetLink subsystem.
      mask init: same as BVH2_App_Layer/BVH2_Appl_Layer/Subsystem/BVH2_Appl_Layer/bl_Pumpoff_Alarm
      settings: DeleteFcn=delete_tlblock(gcbh);  NameChangeFcn=rename_tlblock(gcbh);  OpenFcn=dstabdlg('create','tl_port_dlg',gcbh);  TemplateBlock=tllib/InPort  MemberBlocks=Mixed,NonVirtual,Virtual
      mask Help: eval(['tl_online_help(''Topic'',''',get_param(gcbh,'MaskType'),''')'])
      mask Display: plot([.2 0 .2 .2 .2;.2 1 .8 .8 .2],[.8 .5 .6 .4 .2;.6 .5 .6 .4 .4]);
  ui8_PWM_dc_mat : Subsystem  BlockChoice=Mixed  mask(TL_Inport){data=struct('logdata',struct('maxnumvals',inf,'plotchannels',1,'loggingmode',1,'channels',1),'output',struct('width',1,'name','$B','unit','','type','UInt8','offset',0,'max',200,'min',0,'freeze',1,'lsb',1,'arb',0,'class','GLOBAL','address','','description','','autoscalingmode',1,'lowerheadroom',0,'upperheadroom',1,'headroomunit','bit','show',0,'variable','','scaling','','keepdatatype',1,'castoutput',0),'date',734586.500614051,'message',struct('name','','component','','accessor',''),'virtual',1,'scalingvalid',0), flp_block=none, slscaleparams=, help=|}
      mask help=|
      | InPort block of dSPACE TargetLink.
      |
      | Input signal is read from an external variable and scaled:
      |
      |         y = lsb * u + offset
      mask help:
      | TargetLink Inport block:
      | Defines the input interface of a TargetLink subsystem.
      mask init: same as BVH2_App_Layer/BVH2_Appl_Layer/Subsystem/BVH2_Appl_Layer/bl_Pumpoff_Alarm
      settings: DeleteFcn=delete_tlblock(gcbh);  NameChangeFcn=rename_tlblock(gcbh);  OpenFcn=dstabdlg('create','tl_port_dlg',gcbh);  TemplateBlock=tllib/InPort  MemberBlocks=Mixed,NonVirtual,Virtual
      mask Help: eval(['tl_online_help(''Topic'',''',get_param(gcbh,'MaskType'),''')'])
      mask Display: plot([.2 0 .2 .2 .2;.2 1 .8 .8 .2],[.8 .5 .6 .4 .2;.6 .5 .6 .4 .4]);
  ui8_ResetMatlab : Subsystem  BlockChoice=Mixed  mask(TL_Inport){data=struct('logdata',struct('maxnumvals',inf,'plotchannels',1,'loggingmode',1,'channels',1),'output',struct('width',1,'name','$B','unit','','type','UInt8','offset',0,'max',200,'min',0,'freeze',1,'lsb',1,'arb',0,'class','GLOBAL','address','','description','','autoscalingmode',1,'lowerheadroom',0,'upperheadroom',1,'headroomunit','bit','show',0,'variable','','scaling','','keepdatatype',1,'castoutput',0),'date',734767.594903947,'message',struct('name','','component','','accessor',''),'virtual',1,'scalingvalid',0), flp_block=none, slscaleparams=, help=|}
      mask help=|
      | InPort block of dSPACE TargetLink.
      |
      | Input signal is read from an external variable and scaled:
      |
      |         y = lsb * u + offset
      mask help:
      | TargetLink Inport block:
      | Defines the input interface of a TargetLink subsystem.
      mask init: same as BVH2_App_Layer/BVH2_Appl_Layer/Subsystem/BVH2_Appl_Layer/bl_Pumpoff_Alarm
      settings: DeleteFcn=delete_tlblock(gcbh);  NameChangeFcn=rename_tlblock(gcbh);  OpenFcn=dstabdlg('create','tl_port_dlg',gcbh);  TemplateBlock=tllib/InPort  MemberBlocks=Mixed,NonVirtual,Virtual
      mask Help: eval(['tl_online_help(''Topic'',''',get_param(gcbh,'MaskType'),''')'])
      mask Display: plot([.2 0 .2 .2 .2;.2 1 .8 .8 .2],[.8 .5 .6 .4 .2;.6 .5 .6 .4 .4]);
  ui8_debug_out0 : Subsystem  BlockChoice=Virtual  mask(TL_Outport){data=struct('comment',struct('text','','placement',1),'logdata',struct('maxnumvals',inf,'plotchannels',[],'loggingmode',3,'channels',1),'output',struct('width',1,'name','$B','unit','','type','UInt8','offset',0,'max',NaN,'min',NaN,'freeze',1,'lsb',1,'arb',0,'class','GLOBAL','address','','description','','autoscalingmode',1,'lowerheadroom',0,'upperheadroom',1,'headroomunit','bit','checkmin',0,'checkmax',0,'show',0,'variable','','scaling','','keepdatatype',1,'castoutput',0),'date',734643.687524097,'message',struct('name','','component',''),'virtual',1,'scalingvalid',0), flp_block=none, slscaleparams=, help=|}
      mask help=|
      | OutPort block of dSPACE TargetLink.
      |
      | Input signal is scaled:
      |
      |         y = lsb * u + offset
      mask help:
      | TargetLink Outport block:
      | Defines the output interface of a TargetLink subsystem.
      mask init: same as BVH2_App_Layer/BVH2_Appl_Layer/Subsystem/BVH2_Appl_Layer/bl_Pumpoff_Alarm
      settings: DeleteFcn=delete_tlblock(gcbh);  NameChangeFcn=rename_tlblock(gcbh);  OpenFcn=dstabdlg('create','tl_port_dlg',gcbh);  TemplateBlock=tllib/OutPort  MemberBlocks=Mixed,NonVirtual,Virtual
      mask Help: eval(['tl_online_help(''Topic'',''',get_param(gcbh,'MaskType'),''')'])
      mask Display: plot([0 .2 .2 .8 .8; 1 .8 .8 .8 .8],[.5 .6 .4 .6 .4;.5 .6 .4 .8 .2]);
  ui8_duty_cycle_mat : Subsystem  BlockChoice=Virtual  mask(TL_Outport){data=struct('comment',struct('text','','placement',1),'logdata',struct('maxnumvals',inf,'plotchannels',[],'loggingmode',3,'channels',1),'output',struct('width',1,'name','$B','unit','','type','UInt8','offset',0,'max',NaN,'min',NaN,'freeze',1,'lsb',1,'arb',0,'class','GLOBAL','address','','description','','autoscalingmode',1,'lowerheadroom',0,'upperheadroom',1,'headroomunit','bit','checkmin',0,'checkmax',0,'show',0,'variable','','scaling','','keepdatatype',1,'castoutput',0),'date',734587.454307222,'message',struct('name','','component',''),'virtual',1,'scalingvalid',0), flp_block=none, slscaleparams=, help=|}
      mask help=|
      | OutPort block of dSPACE TargetLink.
      |
      | Input signal is scaled:
      |
      |         y = lsb * u + offset
      mask help:
      | TargetLink Outport block:
      | Defines the output interface of a TargetLink subsystem.
      mask init: same as BVH2_App_Layer/BVH2_Appl_Layer/Subsystem/BVH2_Appl_Layer/bl_Pumpoff_Alarm
      settings: DeleteFcn=delete_tlblock(gcbh);  NameChangeFcn=rename_tlblock(gcbh);  OpenFcn=dstabdlg('create','tl_port_dlg',gcbh);  TemplateBlock=tllib/OutPort  MemberBlocks=Mixed,NonVirtual,Virtual
      mask Help: eval(['tl_online_help(''Topic'',''',get_param(gcbh,'MaskType'),''')'])
      mask Display: plot([0 .2 .2 .8 .8; 1 .8 .8 .8 .8],[.5 .6 .4 .6 .4;.5 .6 .4 .8 .2]);
  ui8_fixed_start_speed_mat : Subsystem  BlockChoice=Mixed  mask(TL_Inport){data=struct('logdata',struct('maxnumvals',inf,'plotchannels',1,'loggingmode',1,'channels',1),'output',struct('width',1,'name','$B','unit','','type','UInt16','offset',0,'max',200,'min',0,'freeze',1,'lsb',1,'arb',0,'class','GLOBAL','address','','description','','autoscalingmode',1,'lowerheadroom',0,'upperheadroom',1,'headroomunit','bit','show',0,'variable','','scaling','','keepdatatype',1,'castoutput',0),'date',734692.64001684,'message',struct('name','','component','','accessor',''),'virtual',1,'scalingvalid',0), flp_block=none, slscaleparams=, help=|}
      mask help=|
      | InPort block of dSPACE TargetLink.
      |
      | Input signal is read from an external variable and scaled:
      |
      |         y = lsb * u + offset
      mask help:
      | TargetLink Inport block:
      | Defines the input interface of a TargetLink subsystem.
      mask init: same as BVH2_App_Layer/BVH2_Appl_Layer/Subsystem/BVH2_Appl_Layer/bl_Pumpoff_Alarm
      settings: DeleteFcn=delete_tlblock(gcbh);  NameChangeFcn=rename_tlblock(gcbh);  OpenFcn=dstabdlg('create','tl_port_dlg',gcbh);  TemplateBlock=tllib/InPort  MemberBlocks=Mixed,NonVirtual,Virtual
      mask Help: eval(['tl_online_help(''Topic'',''',get_param(gcbh,'MaskType'),''')'])
      mask Display: plot([.2 0 .2 .2 .2;.2 1 .8 .8 .2],[.8 .5 .6 .4 .2;.6 .5 .6 .4 .4]);
  Pump_off : Outport
      settings: CopyFcn=if exist('tl_check_ports','file'), tl_check_ports(gcbh); end  NameChangeFcn=if exist('tl_check_ports','file'), tl_check_ports(gcbh); end
  DutyCyclePowerStage : Outport  Port=2
      settings: CopyFcn=if exist('tl_check_ports','file'), tl_check_ports(gcbh); end  NameChangeFcn=if exist('tl_check_ports','file'), tl_check_ports(gcbh); end
  Debug : Outport  Port=3
      settings: CopyFcn=if exist('tl_check_ports','file'), tl_check_ports(gcbh); end  NameChangeFcn=if exist('tl_check_ports','file'), tl_check_ports(gcbh); end
  TemperatureRedAlarm : Outport  Port=4
      settings: CopyFcn=if exist('tl_check_ports','file'), tl_check_ports(gcbh); end  NameChangeFcn=if exist('tl_check_ports','file'), tl_check_ports(gcbh); end
  Motor_stalled : Outport  Port=5
      settings: CopyFcn=if exist('tl_check_ports','file'), tl_check_ports(gcbh); end  NameChangeFcn=if exist('tl_check_ports','file'), tl_check_ports(gcbh); end
  UbatAlarm : Outport  Port=6
      settings: CopyFcn=if exist('tl_check_ports','file'), tl_check_ports(gcbh); end  NameChangeFcn=if exist('tl_check_ports','file'), tl_check_ports(gcbh); end
  PWMin_Alarm : Outport  Port=7
      settings: CopyFcn=if exist('tl_check_ports','file'), tl_check_ports(gcbh); end  NameChangeFcn=if exist('tl_check_ports','file'), tl_check_ports(gcbh); end
  High_Current : Outport  Port=8
      settings: CopyFcn=if exist('tl_check_ports','file'), tl_check_ports(gcbh); end  NameChangeFcn=if exist('tl_check_ports','file'), tl_check_ports(gcbh); end
  TemperatureAlarm : Outport  Port=9
      settings: CopyFcn=if exist('tl_check_ports','file'), tl_check_ports(gcbh); end  NameChangeFcn=if exist('tl_check_ports','file'), tl_check_ports(gcbh); end
  DryRunning : Outport  Port=10
      settings: CopyFcn=if exist('tl_check_ports','file'), tl_check_ports(gcbh); end  NameChangeFcn=if exist('tl_check_ports','file'), tl_check_ports(gcbh); end
  StalledMotorStop : Outport  Port=11
      settings: CopyFcn=if exist('tl_check_ports','file'), tl_check_ports(gcbh); end  NameChangeFcn=if exist('tl_check_ports','file'), tl_check_ports(gcbh); end
  PWMin_Freq_Alarm : Outport  Port=12
      settings: CopyFcn=if exist('tl_check_ports','file'), tl_check_ports(gcbh); end  NameChangeFcn=if exist('tl_check_ports','file'), tl_check_ports(gcbh); end
  PICalarm : Outport  Port=13
      settings: CopyFcn=if exist('tl_check_ports','file'), tl_check_ports(gcbh); end  NameChangeFcn=if exist('tl_check_ports','file'), tl_check_ports(gcbh); end
  wires:
  pwm_input/1 -> ui8_PWM_dc_mat/1(In1)
  bl_Pumpoff_Alarm/1(Out1) -> Pump_off/1
  ui8_duty_cycle_mat/1(Out1) -> DutyCyclePowerStage/1
  Battery Voltage/1 -> ui8_BattVolt_mat/1(In1)
  ui8_BattVolt_mat/1(Out1) -> UbatHandling/1(iUbat)
  RangeAdaption/1(PWMout) -> Saturation/1
  Reset/1 -> ui8_ResetMatlab/1(In1)
  ui8_ResetMatlab/1(Out1) -> UbatHandling/2(iReset), Data Type Conversion2/1, Data Type Conversion4/1, Data Type Conversion5/1, Data Type Conversion7/1, Data Type Conversion6/1, Data Type Conversion3/1, PWM_Detection/3(iReset)
  Speed/1 -> ui16_Speed_mat/1(In1)
  UbatHandling/2(odPumpOff) -> Logical Operator1/2
  UbatHandling/1(odFixedValueSel) -> Logical Operator5/2, Logical Operator7/1
  ui8_Ki_mat/1(Out1) -> Controller/9(Ki)
  Logical Operator1/1 -> Motor_Stalled/1(iMotor_off), Logical Operator3/1
  Saturation/1 -> Controller/8(PWMDirect)
  ui16_Speed_mat/1(Out1) -> Controller/7(Speed), Motor_Stalled/3(iSpeed), Dry_Running/4(iSpeed)
  ui8_debug_out0/1(Out1) -> Debug/1
  ControlLoopMode/1 -> bool_ControlLoopMode/1(In1)
  bool_ControlLoopMode/1(Out1) -> Controller/11(Switch_open_closed)
  PWM_Detection/6(odFixedLowValueSel) -> Controller/1(Fixed_LowDemandSel)
  Temperature1/1 -> ui16_mat_inpTemp/1(In1)
  ui16_mat_inpTemp/1(Out1) -> Data Type Conversion1/1
  bool_CPU_TempRedAlarm/1(Out1) -> TemperatureRedAlarm/1
  Data Type Conversion1/1 -> Temperature_Alarm/1(iTemp)
  Data Type Conversion2/1 -> Temperature_Alarm/2(iReset)
  SpeedDemand/1 -> ui16_Speed_demand_mat/1(In1)
  ui16_Speed_demand_mat/1(Out1) -> Controller/4(SpeedDemand)
  Data Type Conversion3/1 -> Motor_Stalled/2(Reset)
  Speed1/1 -> bool_mat_currAlarm_bldc/1(In1)
  bool_MotorStalled/1(Out1) -> Motor_stalled/1
  UbatHandling/4(oUbat_Alarm_High) -> bool_UbatAlarm/1(In1)
  bool_UbatAlarm/1(Out1) -> UbatAlarm/1
  Controller/2(debug_out0) -> ui8_debug_out0/1(In1)
  bool_PWMin_err_Alarm/1(Out1) -> PWMin_Alarm/1
  Data Type Conversion4/1 -> Current_Analysis_low/2(iReset)
  Current/1 -> ui16_mat_Current/1(In1)
  ui16_mat_Current/1(Out1) -> Dry_Running/3(iCurrent), Current_Analysis_low/1(iCurrent)
  bool_HighCurrentAlarm/1(Out1) -> High_Current/1
  Data Type Conversion5/1 -> Dry_Running/2(iReset)
  MaxSpeed/1 -> ui16_Speed_demand_mat_Max/1(In1)
  MinSpeed/1 -> ui16_Speed_demand_mat_min/1(In1)
  Temperature_Alarm/1(oTempRedAlarm) -> bool_CPU_TempRedAlarm/1(In1)
  bool_CPU_TempAlarm/1(Out1) -> TemperatureAlarm/1
  bool_DryRunningAlarm/1(Out1) -> DryRunning/1
  Temperature_Alarm/3(odPumpOff) -> Logical Operator1/3
  PWM_Freq/1 -> ui16_PWM_Freq_mat/1(In1)
  ui16_PWM_Freq_mat/1(Out1) -> PWM_Detection/1(iPWM_Freq)
  bool_StalledMotorStop/1(Out1) -> StalledMotorStop/1
  Motor_Stalled/1(oMotorStalled) -> bool_StalledMotorStop/1(In1), Logical Operator3/2
  Temperature_Alarm/2(oTempAlarm) -> bool_CPU_TempAlarm/1(In1)
  bool_mat_currAlarm_bldc/1(Out1) -> Current_Analysis_High/1(iAlarm)
  Logical Operator3/1 -> Controller/12(Pump_off)
  Logical Operator5/1 -> Controller/2(Fixed_HighDemand)
  PWM_Detection/1(odFixedValueSel) -> Logical Operator5/1
  ON4/1 -> Controller/3(Fixed_PowerSel)
  PWM_Detection/5(oPWM_Alarm) -> bool_PWMin_err_Alarm/1(In1)
  PWM_Detection/4(oPWM_SC_Alarm) -> bool_PWMin_Freq_err_Alarm/1(In1)
  bool_PWMin_Freq_err_Alarm/1(Out1) -> PWMin_Freq_Alarm/1
  Motor_Stalled/2(oStalledAlarm) -> Logical Operator6/1
  Logical Operator6/1 -> bool_MotorStalled/1(In1)
  ui8_PWM_dc_mat/1(Out1) -> PWM_Detection/2(idPWM), RangeAdaption/1(PWMin), Dry_Running/1(iPWM)
  Gain/1 -> ui8_duty_cycle_mat/1(In1)
  Controller/1(DutyCycle) -> Gain/1
  Data Type Conversion7/1 -> Pic_etat_monitor/2(iReset)
  Pic_etat_monitor/1(oShutoff) -> Logical Operator1/5
  bool_mat_pic_etat/1(Out1) -> Pic_etat_monitor/1(iAlarm)
  PIC_ETAT/1 -> bool_mat_pic_etat/1(In1)
  Dry_Running/1(oDryRunAlarm) -> Dry_RunningAlarm/1(iDryRunAlarm), Logical Operator3/3
  Pic_etat_monitor/2(oAlarm) -> bool_PIC_Alarm/1(In1)
  bool_PIC_Alarm/1(Out1) -> PICalarm/1
  Fixed_start_demand_value/1 -> ui8_fixed_start_speed_mat/1(In1)
  ui16_Speed_demand_mat_min/1(Out1) -> Controller/6(Fixed_LowDemandValue)
  ui16_Speed_demand_mat_Max/1(Out1) -> Controller/5(Fixed_HighDemandValue)
  Logical Operator2/1 -> bl_Pumpoff_Alarm/1(In1), Logical Operator1/1
  PWM_Detection/2(odPumpOff) -> Logical Operator2/1
  Logical Operator7/1 -> Logical Operator2/2
  Ki/1 -> ui8_Ki_mat/1(In1)
  Kp/1 -> ui8_Kp_mat/1(In1)
  ui8_Kp_mat/1(Out1) -> Controller/10(Kp)
  ui8_fixed_start_speed_mat/1(Out1) -> Controller/14(Fixed_Start_DemandValue)
  Start_demand/1 -> bool_start_demand_mat/1(In1)
  bool_start_demand_mat/1(Out1) -> Controller/13(Fixed_Start_Demand)
  DryRunningThreshold/1 -> ui16_dryRun_Thresh/1(In1)
  ui16_dryRun_Thresh/1(Out1) -> Dry_Running/5(iThreshold)
  ui16_Current_Thresh/1(Out1) -> Current_Analysis_low/3(iThreshold)
  Current_Threshold/1 -> ui16_Current_Thresh/1(In1)
  Dry_RunningAlarm/2(oDryRun66) -> bool_DryRunningAlarm/1(In1)
  Dry_RunningAlarm/1(oDryRun55) -> Logical Operator6/3
  Current_Analysis_low/2(oCurrentAlarm) -> bool_HighCurrentAlarm/1(In1)
  Current_Analysis_High/1(oShutoff) -> Logical Operator1/4
  Current_Analysis_High/2(oCurrentAlarm) -> Logical Operator6/2
  Data Type Conversion6/1 -> Current_Analysis_High/2(iReset)
